simulink model "PID_controller"  (R2020b)
settings: Solver=VariableStepAuto  StartTime=0.0  StopTime=10.0  RelTol=1e-3
values from neighbouring files (symbols this model uses):
  kd = 0.15    [variable_declaration.m]
  ki = 500    [variable_declaration.m]
  kp = 21    [variable_declaration.m]
settings Model: Creator=shraddha  LastModifiedBy=shraddha
settings DataIOCC: SaveOutput=off  SaveTime=off

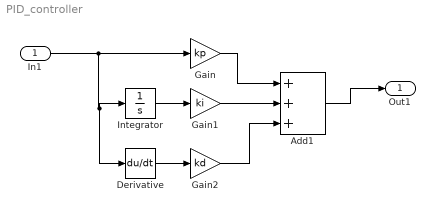
== system PID_controller ==
  In1 : Inport  OutDataTypeStr=double  PortDimensions=1  SampleTime=0
  Add1 : Sum  Inputs=+++
  Derivative : Derivative
  Gain : Gain  Gain=kp
  Gain1 : Gain  Gain=ki
  Gain2 : Gain  Gain=kd
  Integrator : Integrator
  Out1 : Outport  OutDataTypeStr=double  PortDimensions=1  SampleTime=0
  wires:
  Integrator/1 -> Gain1/1
  Gain/1 -> Add1/1
  Gain1/1 -> Add1/2
  In1/1 -> Gain/1, Integrator/1, Derivative/1
  Add1/1 -> Out1/1
  Derivative/1 -> Gain2/1
  Gain2/1 -> Add1/3
